simulink model "Scenariul3_Sarcina_perturbatoare_sim"  (R2025a)
settings: Solver=VariableStepAuto  StartTime=0.0  StopTime=10.0  RelTol=1e-3
values from neighbouring files (symbols this model uses):
  Kd_PD = 0.5    [Scenariul1_Raspuns_treapta.m]    (also in Scenariul2_Referinta_sinusoidala.m = 0.07; Scenariul3_Sarcina_perturbatoare.m = 0.07)
  Kff = 0.07    [Scenariul1_Raspuns_treapta.m]    (also in Scenariul2_Referinta_sinusoidala.m; Scenariul3_Sarcina_perturbatoare.m = -0.03)
  Ki_PI = 1.5    [Scenariul1_Raspuns_treapta.m]    (also in Scenariul2_Referinta_sinusoidala.m = 0.43; Scenariul3_Sarcina_perturbatoare.m = 7)
  Kp_P = 1.5    [Scenariul1_Raspuns_treapta.m]    (also in Scenariul2_Referinta_sinusoidala.m = 0.35; Scenariul3_Sarcina_perturbatoare.m = 0.36)
  Kp_PD = 1    [Scenariul1_Raspuns_treapta.m]    (also in Scenariul2_Referinta_sinusoidala.m = 3.88; Scenariul3_Sarcina_perturbatoare.m = 3.88)
  Kp_PI = 0.4    [Scenariul1_Raspuns_treapta.m]    (also in Scenariul2_Referinta_sinusoidala.m = 0.11; Scenariul3_Sarcina_perturbatoare.m = 0.7)
libraries: simulink x1
settings Model: Creator=luiza  LastModifiedBy=luiza

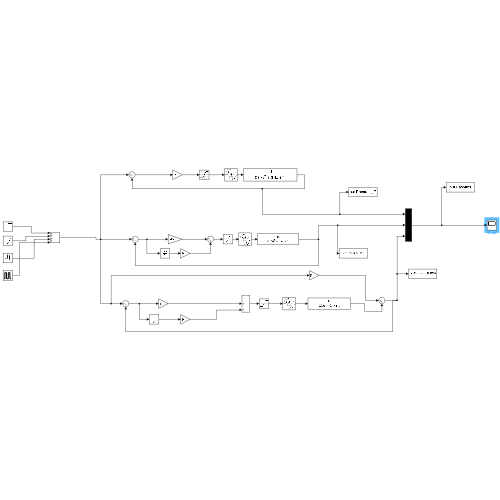
[thumbnail: Simulink's stored preview of the top-level diagram]
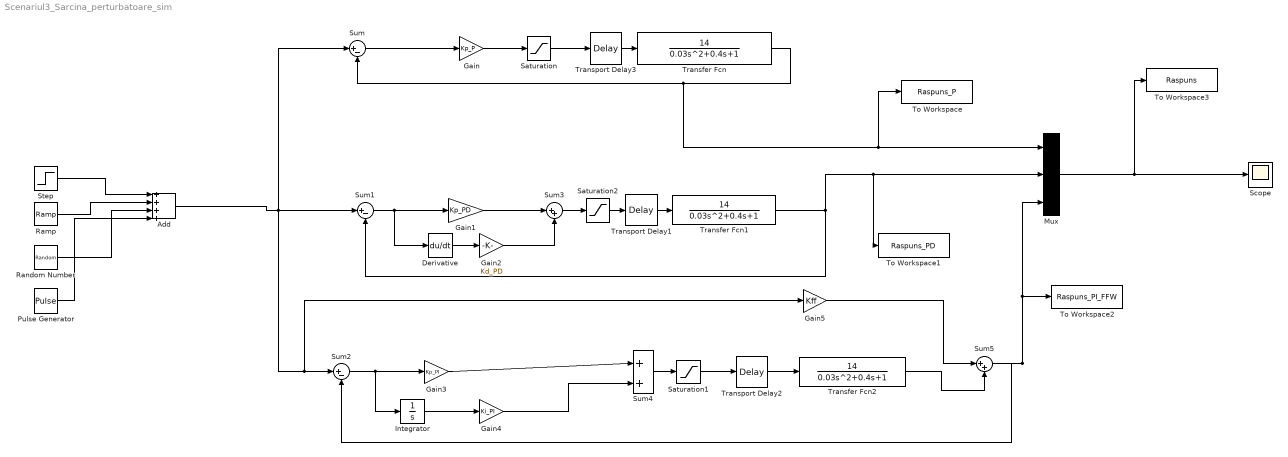
== system Scenariul3_Sarcina_perturbatoare_sim ==
  Add : Sum  Inputs=++++
  Derivative : Derivative
  Gain : Gain  Gain=Kp_P
  Gain1 : Gain  Gain=Kp_PD
  Gain2 : Gain  Gain=Kd_PD
  Gain3 : Gain  Gain=Kp_PI
  Gain4 : Gain  Gain=Ki_PI
  Gain5 : Gain  Gain=Kff
  Integrator : Integrator
  Mux : Mux  Inputs=3
  Pulse Generator : DiscretePulseGenerator  PulseType=Time based  Period=3  PulseWidth=50
  Ramp : simulink/Sources/Ramp  slope=0.5  start=0  InitialOutput=0
  Random Number : RandomNumber  Variance=0.1  SampleTime=0.1
  Saturation : Saturate  UpperLimit=100  LowerLimit=-100
  Saturation1 : Saturate  UpperLimit=100  LowerLimit=-100
  Saturation2 : Saturate  UpperLimit=100  LowerLimit=-100
  Scope : Scope
      settings: ActiveDisplayYMinimum=-178.1214772413569  ActiveDisplayYMaximum=199.13018616684852
  Step : Step  After=10  SampleTime=0
  Sum : Sum  Inputs=|+-
  Sum1 : Sum  Inputs=|+-
  Sum2 : Sum  Inputs=|+-
  Sum3 : Sum  Inputs=|++
  Sum4 : Sum  Inputs=|++
  Sum5 : Sum  Inputs=|++
  To Workspace : ToWorkspace  VariableName=Raspuns_P  SampleTime=-1
  To Workspace1 : ToWorkspace  VariableName=Raspuns_PD  SampleTime=-1
  To Workspace2 : ToWorkspace  VariableName=Raspuns_PI_FFW  SampleTime=-1
  To Workspace3 : ToWorkspace  VariableName=Raspuns  SampleTime=-1
  Transfer Fcn : TransferFcn  Numerator=[14]  Denominator=[0.03 0.4 1]
  Transfer Fcn1 : TransferFcn  Numerator=[14]  Denominator=[0.03 0.4 1]
  Transfer Fcn2 : TransferFcn  Numerator=[14]  Denominator=[0.03 0.4 1]
  Transport Delay1 : TransportDelay  DelayTime=0.05
  Transport Delay2 : TransportDelay  DelayTime=0.05
  Transport Delay3 : TransportDelay  DelayTime=0.05
  wires:
  Sum3/1 -> Saturation2/1
  Derivative/1 -> Gain2/1
  Sum/1 -> Gain/1
  Sum1/1 -> Derivative/1, Gain1/1
  Transport Delay3/1 -> Transfer Fcn/1
  Mux/1 -> To Workspace3/1, Scope/1
  Gain1/1 -> Sum3/1
  Integrator/1 -> Gain4/1
  Sum2/1 -> Integrator/1, Gain3/1
  Gain4/1 -> Sum4/2
  Saturation/1 -> Transport Delay3/1
  Gain2/1 -> Sum3/2
  Gain/1 -> Saturation/1
  Transfer Fcn1/1 -> Sum1/2, To Workspace1/1, Mux/2
  Sum4/1 -> Saturation1/1
  Transport Delay1/1 -> Transfer Fcn1/1
  Gain3/1 -> Sum4/1
  Saturation2/1 -> Transport Delay1/1
  Transfer Fcn/1 -> To Workspace/1, Mux/1, Sum/2
  Saturation1/1 -> Transport Delay2/1
  Ramp/1 -> Add/2
  Random Number/1 -> Add/3
  Add/1 -> Gain5/1, Sum2/1, Sum/1, Sum1/1
  Pulse Generator/1 -> Add/4
  Transport Delay2/1 -> Transfer Fcn2/1
  Gain5/1 -> Sum5/1
  Transfer Fcn2/1 -> Sum5/2
  Sum5/1 -> Sum2/2, Mux/3, To Workspace2/1
  Step/1 -> Add/1
